simulink model "Control_system_v5"  (R2024b)
settings: Solver=FixedStepDiscrete  StartTime=0.0  StopTime=1000  FixedStep=1  RelTol=1e-3
undefined symbols (not defined in the file): C, Cj, Cq, Cw, D, Dj, Dq, Dw, G, Gq, Gw, H, Hq, Hw, I_a, K, start_time, start_time_QW, Vk, Wk, x_eq, y_eq
settings Model: Creator=54238  LastModifiedBy=54238
settings DebuggingCC: AlgebraicLoopMsg=none

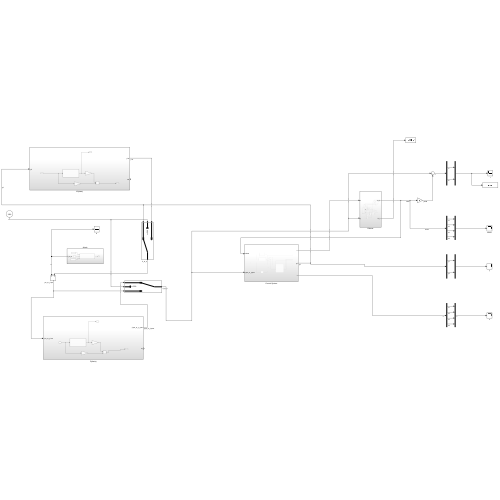
[thumbnail: Simulink's stored preview of the top-level diagram]
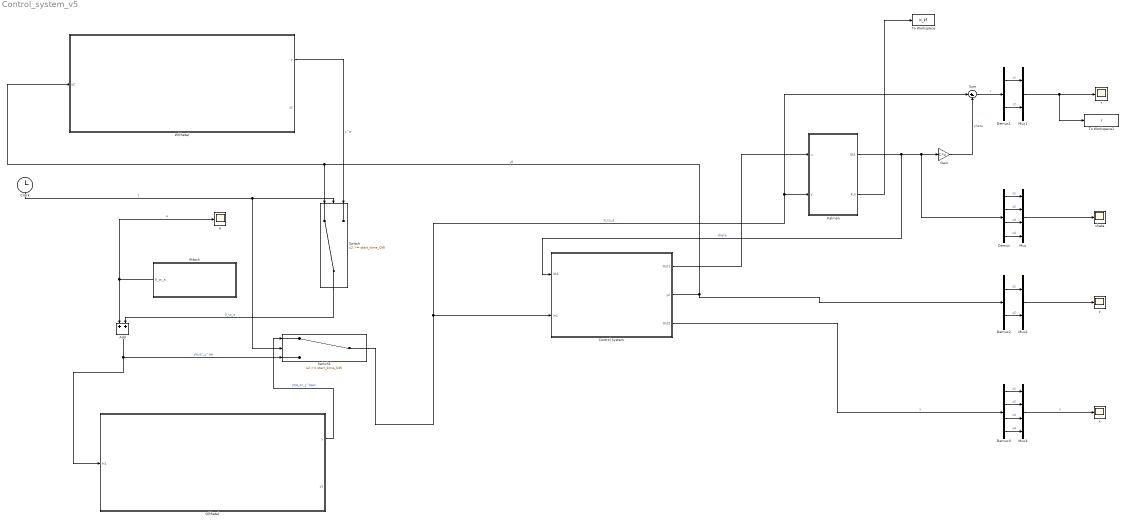
== system Control_system_v5 ==
  Add : Sum
  Attack : Subsystem
  Clock : Clock
  Control System : Subsystem
  Demux : Demux
  Demux1 : Demux  Outputs=2
  Demux2 : Demux  Outputs=2
  Demux3 : Demux
  Gain : Gain  Gain=C  Multiplication=Matrix(K*u)
  Kalman : Subsystem
  Mux : Mux
  Mux1 : Mux  Inputs=2
  Mux2 : Mux  Inputs=2
  Mux3 : Mux
  Q(theta) : Subsystem
  Sum : Sum  Inputs=|+-
  Switch : Switch  Threshold=start_time_QW  SaturateOnIntegerOverflow=off  InputSameDT=off
  Switch1 : Switch  Threshold=start_time_QW  SaturateOnIntegerOverflow=off  InputSameDT=off
  To Workspace : ToWorkspace  VariableName=K_kf  SampleTime=-1
  To Workspace1 : ToWorkspace  VariableName=r  SaveFormat=Timeseries  SampleTime=-1
  W(theta) : Subsystem
  a : Scope
  r : Scope
  x : Scope
  xheta : Scope
  y : Scope
  wires:
  Control System/1(Out1) -> Kalman/1(u)
  Gain/1 -> Sum/2  "yheta"
  Kalman/2(K_k) -> To Workspace/1
  Kalman/1(Xk1) -> Control System/1(Xk1), Demux/1, Gain/1  "xheta"
  Mux/1 -> xheta/1
  Demux/4 -> Mux/4  "x4"
  Sum/1 -> Demux1/1  "r"
  Mux1/1 -> To Workspace1/1, r/1
  Demux/1 -> Mux/1  "x1"
  Demux/2 -> Mux/2  "x2"
  Demux/3 -> Mux/3  "x3"
  Demux1/1 -> Mux1/1  "r1"
  Demux1/2 -> Mux1/2  "r2"
  Demux2/1 -> Mux2/1  "y1"
  Mux2/1 -> y/1
  Demux2/2 -> Mux2/2  "y2"
  Control System/2(y2) -> Switch/1, W(theta)/1(y2), Demux2/1  "y0"
  Demux3/4 -> Mux3/4  "x4"
  Demux3/1 -> Mux3/1  "x1"
  Control System/3(Out2) -> Demux3/1  "x"
  Demux3/2 -> Mux3/2  "x2"
  Demux3/3 -> Mux3/3  "x3"
  Mux3/1 -> x/1  "x"
  Attack/1(0_to_a) -> Add/1, a/1  "a"
  Add/1 -> Switch1/3, Q(theta)/1(In1)  "yw_or_y^qw"
  Clock/1 -> Switch1/2, Switch/2  "t"
  Switch/1 -> Add/2  "0_to_a"
  Switch1/1 -> Control System/2(In1), Sum/1, Kalman/2(y)  "0_to_a"
  Q(theta)/1(y) -> Switch1/1  "yqw_or_y^qaw"
  W(theta)/1(y) -> Switch/3  "y^w"

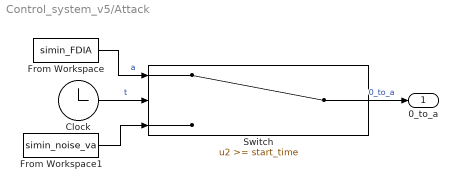
== system Control_system_v5/Attack ==
  Clock : Clock
  From Workspace : FromWorkspace  VariableName=simin_FDIA  SampleTime=-1
  From Workspace1 : FromWorkspace  VariableName=simin_noise_va  SampleTime=-1
  Switch : Switch  Threshold=start_time  SaturateOnIntegerOverflow=off  InputSameDT=off
  0_to_a : Outport
  wires:
  From Workspace1/1 -> Switch/3
  Clock/1 -> Switch/2  "t"
  From Workspace/1 -> Switch/1  "a"
  Switch/1 -> 0_to_a/1  "0_to_a"

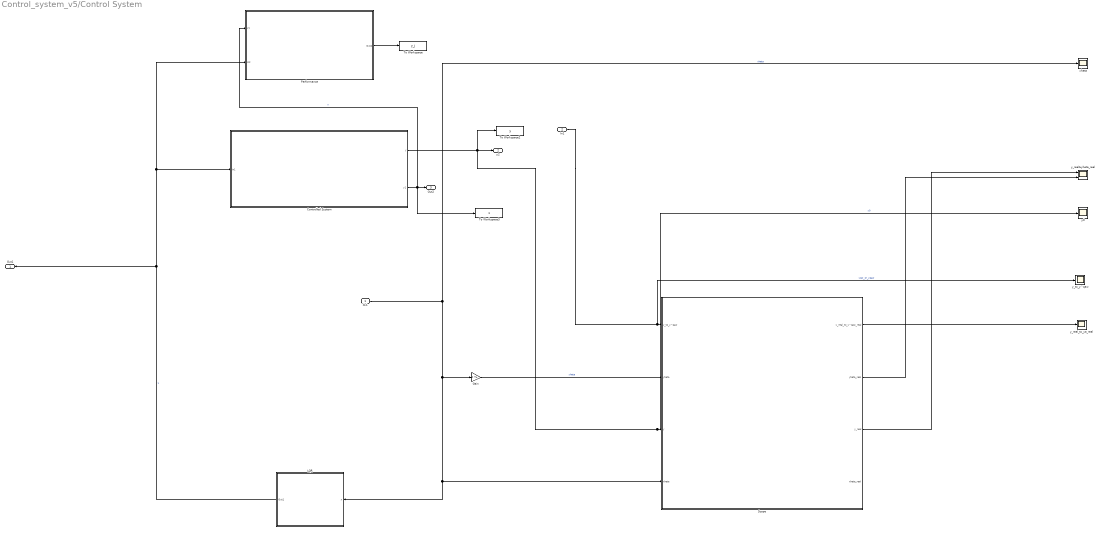
== system Control_system_v5/Control System ==
  Xk1 : Inport
  In1 : Inport  Port=2
  Controlled System : Subsystem
  Gain : Gain  Gain=C  Multiplication=Matrix(K*u)
  LQR : Subsystem
  Performance : Subsystem
  Scope : Subsystem
  To Workspace : ToWorkspace  VariableName=y_j  SaveFormat=Timeseries  SampleTime=-1
  To Workspace2 : ToWorkspace  VariableName=y  SaveFormat=Timeseries  SampleTime=-1
  To Workspace3 : ToWorkspace  VariableName=x  SaveFormat=Timeseries  SampleTime=-1
  xheta : Scope
  y0 : Scope
  y_real&yheta_real : Scope  NumInputPorts=2
  y_real_to_ya_real : Scope
  y_to_y^qaw : Scope
  Out1 : Outport  PortDimensions=[2,1]
  y2 : Outport  Port=2
  Out2 : Outport  Port=3
  wires:
  LQR/1(Out1) -> Performance/2(In2), Controlled System/1(In1), Out1/1  "u"
  Xk1/1 -> Scope/4(xheta), LQR/1(x), Gain/1, xheta/1  "xheta"
  Controlled System/1(y) -> y0/1, Scope/3(y), To Workspace2/1, y2/1  "y0"
  In1/1 -> y_to_y^qaw/1, Scope/1(y_to_y^qaw)  "yqw_or_yqaw"
  Gain/1 -> Scope/2(yheta)  "yheta"
  Scope/3(y_real) -> y_real&yheta_real/1
  Scope/2(yheta_real) -> y_real&yheta_real/2
  Scope/1(y_real_to_y^qaw_real) -> y_real_to_ya_real/1
  Controlled System/2(y1) -> To Workspace3/1, Performance/1(y1), Out2/1  "x"
  Performance/1(Out2) -> To Workspace/1

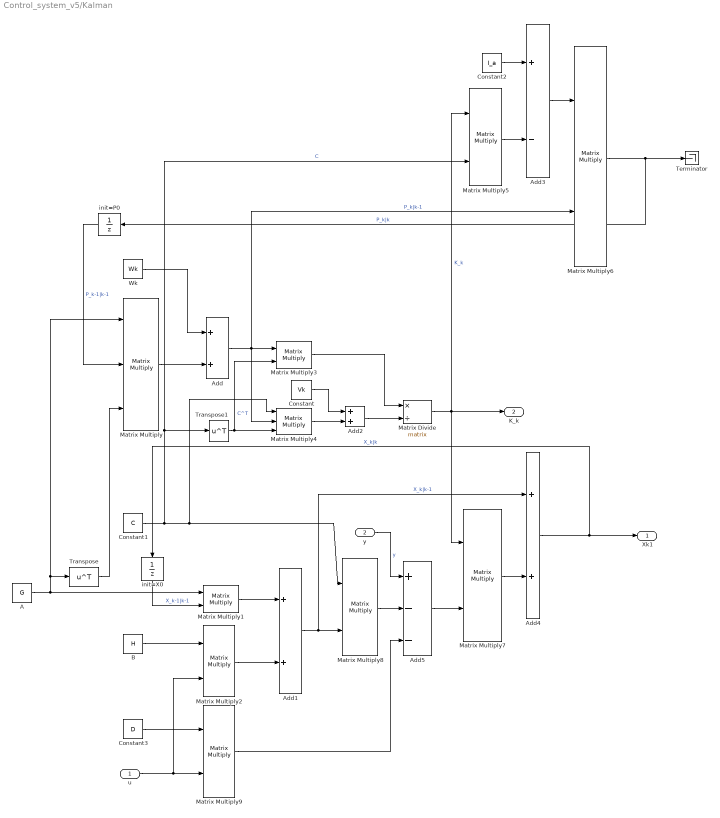
== system Control_system_v5/Kalman ==
  u : Inport  PortDimensions=[2,1]
  y : Inport  Port=2  PortDimensions=[2,1]
  A : Constant  Value=G
  Add{,1..2,4} (4 alike) : Sum
  Add3 : Sum  Inputs=+-
  Add5 : Sum  Inputs=+--
  B : Constant  Value=H
  Constant : Constant  Value=Vk
  Constant1 : Constant  Value=C
  Constant2 : Constant  Value=I_a
  Constant3 : Constant  Value=D
  Matrix Divide : Product  Inputs=*/  Multiplication=Matrix(*)
  Matrix Multiply : Product  Inputs=3  Multiplication=Matrix(*)
  Matrix Multiply{1..3,5..9} (8 alike) : Product  Multiplication=Matrix(*)
  Matrix Multiply4 : Product  Inputs=3  Multiplication=Matrix(*)
  Terminator : Terminator
  Transpose : Math  Operator=transpose  SignedPower=on  RndMeth=Zero
  Transpose1 : Math  Operator=transpose
  Wk : Constant  Value=Wk
  init=P0 : UnitDelay  SampleTime=-1  StateName=p0  HasFrameUpgradeWarning=on
  init=X0 : UnitDelay  InitialCondition=[5;5;2.044;1.399]  SampleTime=-1  HasFrameUpgradeWarning=on
  Xk1 : Outport  PortDimensions=[4,1]
  K_k : Outport  Port=2
  wires:
  Matrix Multiply2/1 -> Add1/2
  Add5/1 -> Matrix Multiply7/2
  Matrix Multiply6/1 -> Terminator/1, init=P0/1  "P_k|k"
  Constant1/1 -> Matrix Multiply4/1, Matrix Multiply8/1, Matrix Multiply5/2, Transpose1/1  "C"
  Add4/1 -> Xk1/1, init=X0/1  "X_k|k"
  Constant/1 -> Add2/1
  A/1 -> Matrix Multiply/1, Transpose/1, Matrix Multiply1/1
  Add1/1 -> Matrix Multiply8/2, Add4/1  "X_k|k-1"
  Constant2/1 -> Add3/1
  Add/1 -> Matrix Multiply3/1, Matrix Multiply4/2, Matrix Multiply6/2  "P_k|k-1"
  Add3/1 -> Matrix Multiply6/1
  init=X0/1 -> Matrix Multiply1/2  "X_k-1|k-1"
  Transpose/1 -> Matrix Multiply/3
  Matrix Multiply7/1 -> Add4/2
  init=P0/1 -> Matrix Multiply/2  "P_k-1|k-1"
  Matrix Multiply/1 -> Add/2
  Transpose1/1 -> Matrix Multiply4/3, Matrix Multiply3/2  "C^T"
  Wk/1 -> Add/1
  y/1 -> Add5/1  "y"
  Matrix Multiply5/1 -> Add3/2
  Matrix Divide/1 -> Matrix Multiply5/1, K_k/1, Matrix Multiply7/1  "K_k"
  u/1 -> Matrix Multiply2/2, Matrix Multiply9/2
  Matrix Multiply1/1 -> Add1/1
  Add2/1 -> Matrix Divide/2
  Matrix Multiply4/1 -> Add2/2
  Constant3/1 -> Matrix Multiply9/1
  Matrix Multiply8/1 -> Add5/2
  B/1 -> Matrix Multiply2/1
  Matrix Multiply9/1 -> Add5/3
  Matrix Multiply3/1 -> Matrix Divide/1

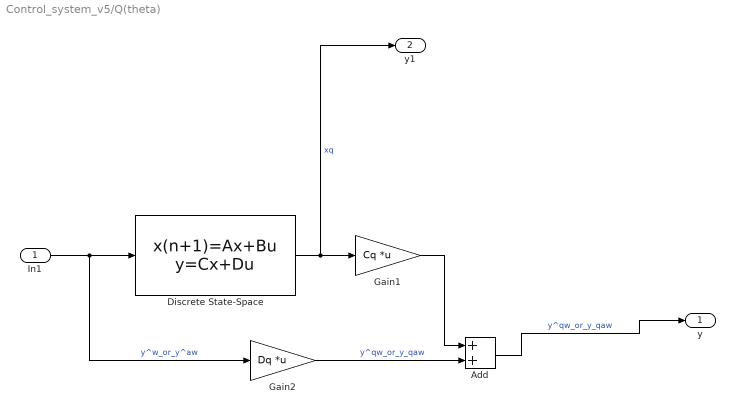
== system Control_system_v5/Q(theta) ==
  In1 : Inport
  Add : Sum
  Discrete State-Space : DiscreteStateSpace  A=Gq  B=Hq  C=[1 0 0 0;0 1 0 0;0 0 1 0;0 0 0 1]  D=[0 0;0 0;0 0;0 0]  InitialCondition=[0 0 0 0]  SampleTime=-1
  Gain1 : Gain  Gain=Cq  Multiplication=Matrix(K*u)
  Gain2 : Gain  Gain=Dq  Multiplication=Matrix(K*u)
  y : Outport
  y1 : Outport  Port=2
  wires:
  Discrete State-Space/1 -> y1/1, Gain1/1  "xq"
  In1/1 -> Gain2/1, Discrete State-Space/1  "y^w_or_y^aw"
  Gain1/1 -> Add/1
  Gain2/1 -> Add/2  "y^qw_or_y_qaw"
  Add/1 -> y/1  "y^qw_or_y_qaw"

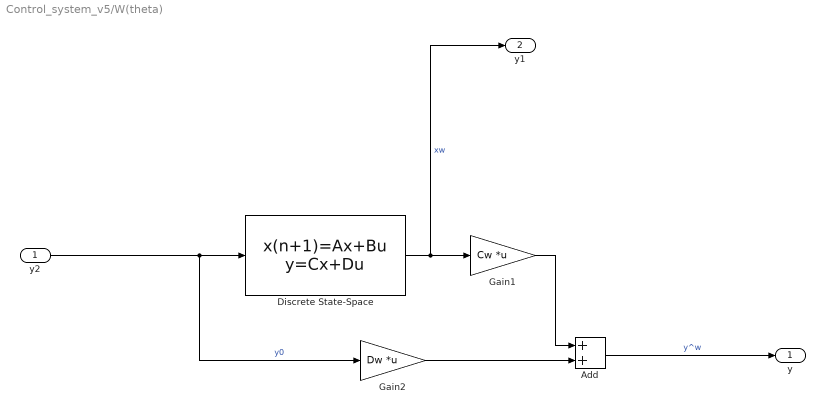
== system Control_system_v5/W(theta) ==
  y2 : Inport
  Add : Sum
  Discrete State-Space : DiscreteStateSpace  A=Gw  B=Hw  C=[1 0 0 0;0 1 0 0;0 0 1 0;0 0 0 1]  D=[0 0;0 0;0 0;0 0]  InitialCondition=[0 0 0 0]  SampleTime=-1
  Gain1 : Gain  Gain=Cw  Multiplication=Matrix(K*u)
  Gain2 : Gain  Gain=Dw  Multiplication=Matrix(K*u)
  y : Outport
  y1 : Outport  Port=2
  wires:
  Discrete State-Space/1 -> y1/1, Gain1/1  "xw"
  y2/1 -> Gain2/1, Discrete State-Space/1  "y0"
  Gain1/1 -> Add/1
  Gain2/1 -> Add/2
  Add/1 -> y/1  "y^w"

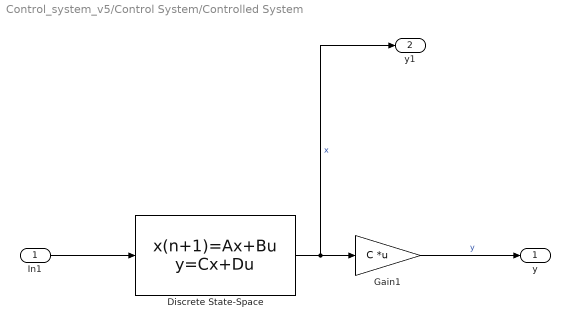
== system Control_system_v5/Control System/Controlled System ==
  In1 : Inport
  Discrete State-Space : DiscreteStateSpace  A=G  B=H  C=[1 0 0 0;0 1 0 0;0 0 1 0;0 0 0 1]  D=[0 0;0 0;0 0;0 0]  InitialCondition=[0 0 0 0]  SampleTime=-1
  Gain1 : Gain  Gain=C  Multiplication=Matrix(K*u)
  y : Outport
  y1 : Outport  Port=2
  wires:
  Gain1/1 -> y/1  "y"
  Discrete State-Space/1 -> y1/1, Gain1/1  "x"
  In1/1 -> Discrete State-Space/1

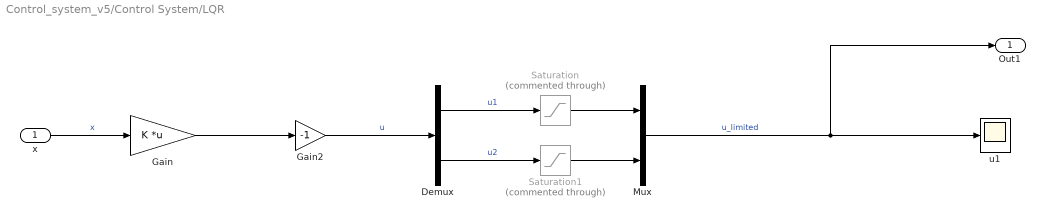
== system Control_system_v5/Control System/LQR ==
  x : Inport
  Demux : Demux  Outputs=2
  Gain : Gain  Gain=K  Multiplication=Matrix(K*u)
  Gain2 : Gain  Gain=-1
  Mux : Mux  Inputs=2
  Saturation : Saturate  Commented=through  UpperLimit=0.999  LowerLimit=-0.999
  Saturation1 : Saturate  Commented=through  UpperLimit=1.005  LowerLimit=-1.005
  u1 : Scope
  Out1 : Outport  PortDimensions=[2,1]
  wires:
  Saturation/1 -> Mux/1
  x/1 -> Gain/1  "x"
  Demux/1 -> Saturation/1  "u1"
  Mux/1 -> Out1/1, u1/1  "u_limited"
  Demux/2 -> Saturation1/1  "u2"
  Saturation1/1 -> Mux/2
  Gain/1 -> Gain2/1
  Gain2/1 -> Demux/1  "u"

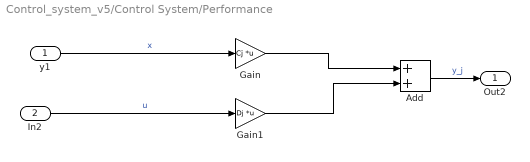
== system Control_system_v5/Control System/Performance ==
  y1 : Inport
  In2 : Inport  Port=2
  Add : Sum
  Gain : Gain  Gain=Cj  Multiplication=Matrix(K*u)
  Gain1 : Gain  Gain=Dj  Multiplication=Matrix(K*u)
  Out2 : Outport
  wires:
  In2/1 -> Gain1/1  "u"
  y1/1 -> Gain/1  "x"
  Gain/1 -> Add/1
  Add/1 -> Out2/1  "y_j"
  Gain1/1 -> Add/2

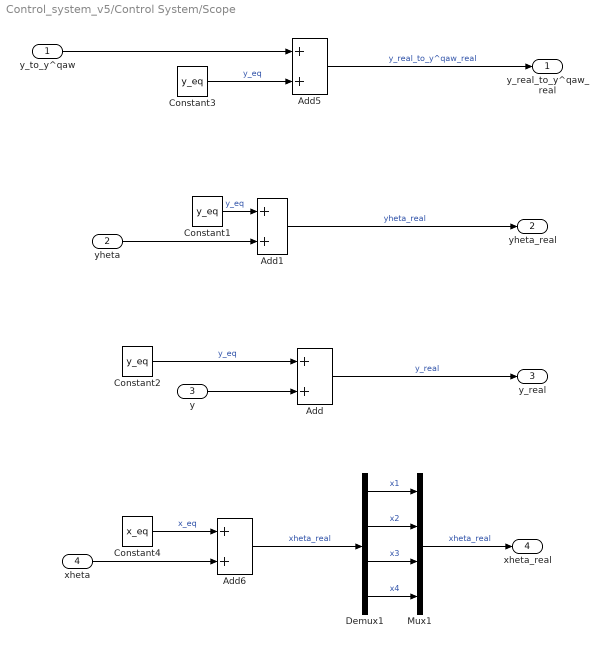
== system Control_system_v5/Control System/Scope ==
  y_to_y^qaw : Inport
  yheta : Inport  Port=2
  y : Inport  Port=3
  xheta : Inport  Port=4
  Add{,1,5..6} (4 alike) : Sum
  Constant1 : Constant  Value=y_eq  VectorParams1D=off
  Constant2 : Constant  Value=y_eq  VectorParams1D=off
  Constant3 : Constant  Value=y_eq  VectorParams1D=off
  Constant4 : Constant  Value=x_eq  VectorParams1D=off
  Demux1 : Demux
  Mux1 : Mux
  y_real_to_y^qaw_real : Outport
  yheta_real : Outport  Port=2
  y_real : Outport  Port=3
  xheta_real : Outport  Port=4
  wires:
  Demux1/1 -> Mux1/1  "x1"
  Constant4/1 -> Add6/1  "x_eq"
  Constant2/1 -> Add/1  "y_eq"
  Constant3/1 -> Add5/2  "y_eq"
  Add6/1 -> Demux1/1  "xheta_real"
  Add5/1 -> y_real_to_y^qaw_real/1  "y_real_to_y^qaw_real"
  Constant1/1 -> Add1/1  "y_eq"
  Demux1/3 -> Mux1/3  "x3"
  Demux1/2 -> Mux1/2  "x2"
  Demux1/4 -> Mux1/4  "x4"
  Add1/1 -> yheta_real/1  "yheta_real"
  yheta/1 -> Add1/2
  y/1 -> Add/2
  y_to_y^qaw/1 -> Add5/1
  Mux1/1 -> xheta_real/1  "xheta_real"
  Add/1 -> y_real/1  "y_real"
  xheta/1 -> Add6/2
